simulink model "RRRRR_controller"  (R2020a)
settings: Solver=ode3  StartTime=0.0  StopTime=10  RelTol=1e-3
libraries: roblocks x4
settings Model: Creator=yrza  LastModifiedBy=Anuar

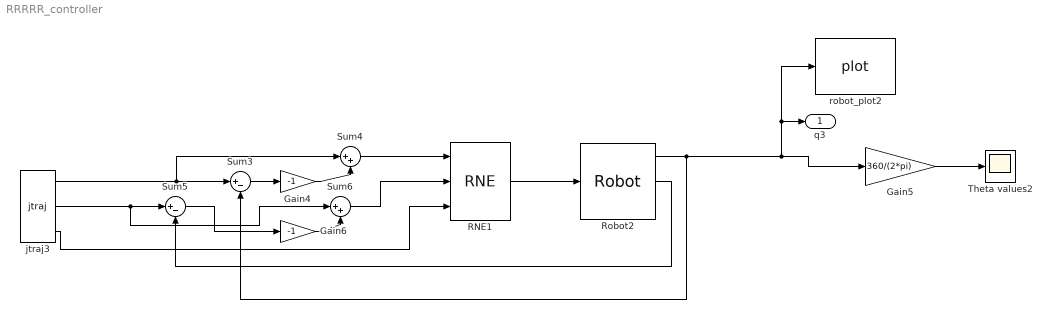
== system RRRRR_controller ==
  Gain4 : Gain  Gain=-1
  Gain5 : Gain  Gain=360/(2*pi)
  Gain6 : Gain  Gain=-1
  RNE1 : roblocks/Arm/RNE  robot=planar  grav=[0 0 9.81]
  Robot2 : roblocks/Arm/Robot  robot=planar  q0=[0 0 0 0 0]
  Sum3 : Sum  Inputs=|+-
  Sum4 : Sum  Inputs=|++
  Sum5 : Sum  Inputs=|+-
  Sum6 : Sum  Inputs=|++
  Theta values2 : Scope
  jtraj3 : roblocks/Toolbox/jtraj  q0=[0 0 0 0 0]  qf=[pi/2 -pi/4 -pi/4 -pi/4 -pi/4]  tmax=2.02  ts=0.02
  robot_plot2 : roblocks/Arm/plot  robot=planar  fps=5  holdplot=on
  q3 : Outport
  wires:
  RNE1/1 -> Robot2/1
  Gain5/1 -> Theta values2/1
  Robot2/1 -> Sum3/2, robot_plot2/1, q3/1, Gain5/1
  jtraj3/1 -> Sum4/1, Sum3/1
  jtraj3/3 -> RNE1/3
  Sum4/1 -> RNE1/1
  Sum3/1 -> Gain4/1
  Gain4/1 -> Sum4/2
  Robot2/2 -> Sum5/2
  jtraj3/2 -> Sum6/1, Sum5/1
  Gain6/1 -> Sum6/2
  Sum5/1 -> Gain6/1
  Sum6/1 -> RNE1/2
